simulink model "T2_Linarized_2_dof_Helicopter"  (R2023a)
settings: Solver=ode4  StartTime=0.0  StopTime=inf  FixedStep=0.1  RelTol=1e-3
values from neighbouring files (symbols this model uses):
  Ac = [0,0,1,0 ... (first row only)    [Linerized_Parameters.m]
  Bc = [0,0 ... (first row only)    [Linerized_Parameters.m]
  p_op = pi/2    (= 1.57079632679)    [Linerized_Parameters.m]
  t_op = (-10*pi)/180    (= -0.174532925199)    [Linerized_Parameters.m]
  V_mp_op = (K_yy* m_heli*g*cos(t_op)*l_cm  )/((K_yy*K_pp-K_yp*K_py))    [Linerized_Parameters.m]
  V_my_op = (K_yp* V_mp_op)/K_yy    [Linerized_Parameters.m]
  wp_op = 0    [Linerized_Parameters.m]
  wt_op = 0    [Linerized_Parameters.m]
libraries: realtime_pacer_lib x1
settings Model: Creator=aleho  LastModifiedBy=aleho

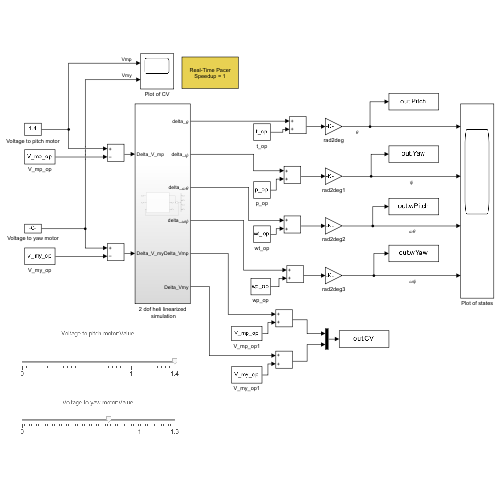
[thumbnail: Simulink's stored preview of the top-level diagram]
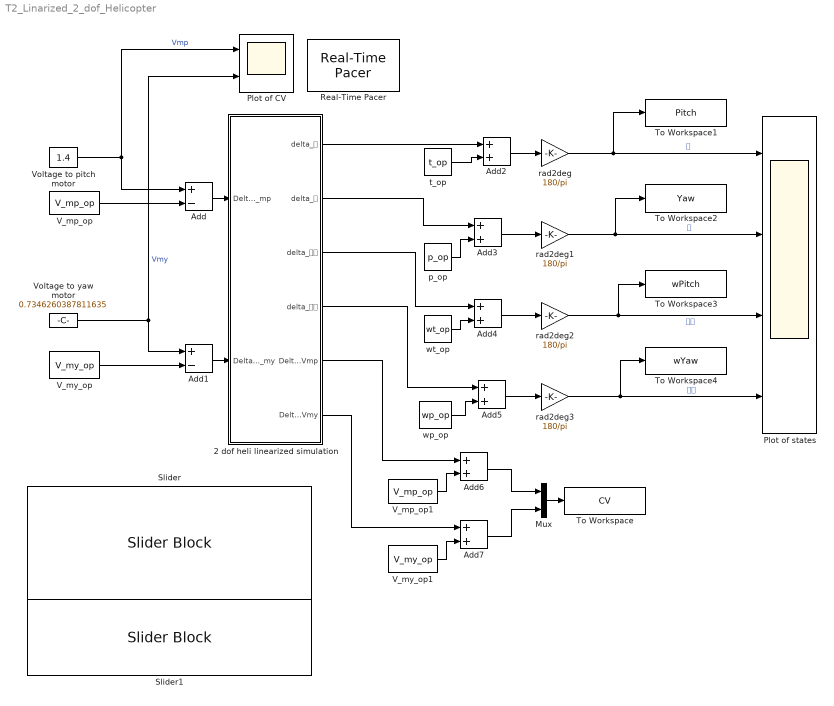
== system T2_Linarized_2_dof_Helicopter ==
  2 dof heli linearized simulation : Subsystem
  Add : Sum  Inputs=+-
  Add1 : Sum  Inputs=+-
  Add{2..7} (6 alike) : Sum
  Mux : Mux  Inputs=2
  Plot of CV : Scope  NumInputPorts=2
  Plot of states : Scope  NumInputPorts=4
  Real-Time Pacer : realtime_pacer_lib/Real-Time Pacer  simTimePerRealTime=1
  Slider : SliderBlock  ScaleMax=1.4  TickInterval=1
  Slider1 : SliderBlock  ScaleMax=1.3  TickInterval=1
  To Workspace : ToWorkspace  VariableName=CV  SaveFormat=Timeseries  SampleTime=-1
  To Workspace1 : ToWorkspace  VariableName=Pitch  SaveFormat=Timeseries  SampleTime=-1
  To Workspace2 : ToWorkspace  VariableName=Yaw  SaveFormat=Timeseries  SampleTime=-1
  To Workspace3 : ToWorkspace  VariableName=wPitch  SaveFormat=Timeseries  SampleTime=-1
  To Workspace4 : ToWorkspace  VariableName=wYaw  SaveFormat=Timeseries  SampleTime=-1
  V_mp_op : Constant  Value=V_mp_op
  V_mp_op1 : Constant  Value=V_mp_op
  V_my_op : Constant  Value=V_my_op
  V_my_op1 : Constant  Value=V_my_op
  Voltage to pitch motor : Constant  Value=1.4
  Voltage to yaw motor : Constant  Value=0.7346260387811635
  p_op : Constant  Value=p_op
  rad2deg{,1..3} (4 alike) : Gain  Gain=180/pi
  t_op : Constant  Value=t_op
  wp_op : Constant  Value=wp_op
  wt_op : Constant  Value=wt_op
  wires:
  Voltage to pitch motor/1 -> Plot of CV/1, Add/1  "Vmp"
  Voltage to yaw motor/1 -> Plot of CV/2, Add1/1  "Vmy"
  Add/1 -> 2 dof heli linearized simulation/1(Delta_V_mp)
  V_mp_op/1 -> Add/2
  Add1/1 -> 2 dof heli linearized simulation/2(Delta_V_my)
  V_my_op/1 -> Add1/2
  t_op/1 -> Add2/2
  p_op/1 -> Add3/2
  wp_op/1 -> Add5/2
  wt_op/1 -> Add4/2
  2 dof heli linearized simulation/1(delta_𝜃) -> Add2/1
  2 dof heli linearized simulation/2(delta_𝜓) -> Add3/1
  2 dof heli linearized simulation/3(delta_𝜔𝜃) -> Add4/1
  2 dof heli linearized simulation/4(delta_𝜔𝜓) -> Add5/1
  rad2deg/1 -> To Workspace1/1, Plot of states/1  "𝜃"
  Add2/1 -> rad2deg/1
  rad2deg1/1 -> To Workspace2/1, Plot of states/2  "𝜓"
  Add3/1 -> rad2deg1/1
  rad2deg2/1 -> To Workspace3/1, Plot of states/3  "𝜔𝜃"
  Add4/1 -> rad2deg2/1
  rad2deg3/1 -> To Workspace4/1, Plot of states/4  "𝜔𝜓"
  Add5/1 -> rad2deg3/1
  2 dof heli linearized simulation/5(Delta_Vmp) -> Add6/1
  Add6/1 -> Mux/1
  2 dof heli linearized simulation/6(Delta_Vmy) -> Add7/1
  Add7/1 -> Mux/2
  V_mp_op1/1 -> Add6/2
  V_my_op1/1 -> Add7/2
  Mux/1 -> To Workspace/1

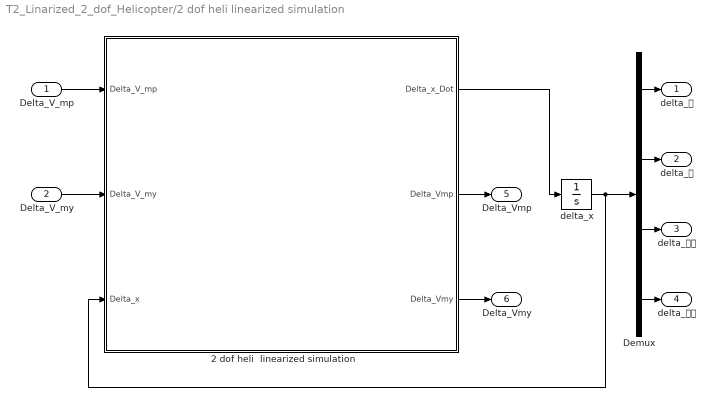
== system T2_Linarized_2_dof_Helicopter/2 dof heli linearized simulation ==
  Delta_V_mp : Inport
  Delta_V_my : Inport  Port=2
  2 dof heli  linearized simulation : MATLAB Function  TreatAsAtomicUnit=on
  Demux : Demux
  delta_x : Integrator  InitialCondition=[-45*pi/180,pi/2,0,0]  LimitOutput=on  UpperSaturationLimit=[45*pi/180,pi,2,2]  LowerSaturationLimit=[-45*pi/180,0,-2,-2]
  delta_𝜃 : Outport
  delta_𝜓 : Outport  Port=2
  delta_𝜔𝜃 : Outport  Port=3
  delta_𝜔𝜓 : Outport  Port=4
  Delta_Vmp : Outport  Port=5
  Delta_Vmy : Outport  Port=6
  wires:
  Delta_V_mp/1 -> 2 dof heli  linearized simulation/1(Delta_V_mp)
  delta_x/1 -> 2 dof heli  linearized simulation/3(Delta_x), Demux/1
  Demux/1 -> delta_𝜃/1
  Demux/4 -> delta_𝜔𝜓/1
  Demux/3 -> delta_𝜔𝜃/1
  Demux/2 -> delta_𝜓/1
  2 dof heli  linearized simulation/1(Delta_x_Dot) -> delta_x/1
  Delta_V_my/1 -> 2 dof heli  linearized simulation/2(Delta_V_my)
  2 dof heli  linearized simulation/2(Delta_Vmp) -> Delta_Vmp/1
  2 dof heli  linearized simulation/3(Delta_Vmy) -> Delta_Vmy/1

== matlab function T2_Linarized_2_dof_Helicopter/2 dof heli linearized simulation/2 dof heli  linearized simulation ==
  data: Delta_V_mp input; Delta_V_my input; Delta_x input; Bc parameter; Ac parameter; Delta_x_Dot output; Delta_Vmp output; Delta_Vmy output
function [Delta_x_Dot, Delta_Vmp,Delta_Vmy] = linear_model(Delta_V_mp,Delta_V_my,Delta_x, Bc, Ac)

Delta_Vmp = Delta_V_mp;
Delta_Vmy = Delta_V_my;

% Linear state space model equation
Delta_u = [Delta_V_mp ;Delta_V_my];
Delta_x_Dot = Ac*Delta_x + Bc*Delta_u;
